simulink model "model_cnn"  (R2020a)
settings: Solver=VariableStepAuto  StartTime=0.0  StopTime=1e6/fs  RelTol=1e-3
PreLoadFcn:
  | setup_imports;
  | %dense2_numerictype = fixdt(1,18,10);
  | %conv1_numerictype = fixdt(1,18,21);
InitFcn:
  | % Intermediate signal dimensions
  | input_dim = [1, 2, 128];
  | layer1_dim = hInterConvLayerDims([1,3,1,64],input_dim,1); % dims : [C,H,W]
  | layer2_dim = hInterConvLayerDims([2,3,64,16],layer1_dim,1);% dims : [C,H,W]
  | layer3_dim = [1,128];
  | 
  | % Conv Layer 1 dimensions
  | conv1_dims = struct(...
  |     'input_dim',    input_dim,...       input_dim = C,H,W
  |     'filter_dim',   [1, 3, 1, 64],...  filter_dim = K,J,C,N
  |     'stride',       1,...
  |     'row_output',   3,...
  |     'output_dim',   layer1_dim);
  | 
  | % Conv Layer 2 dimensions
  | conv2_dims = struct(...
  |     'input_dim',    layer1_dim,...      input = C,H.W
  |     'filter_dim',   [2, 3, 64, 16],...  filter_dim = K,J,C,N
  |     'stride',       1,...
  |     'row_output',   2*3*64,...
  |     'output_dim',   layer2_dim);
  | 
  | % Dense Layer 1 dimensions
  | dense1_dims = struct(...
  |     'input_dim',    layer2_dim,...      input = C,H,W
  |     'weight_dim',   [1984, 128],...     weight_dim = H,W
  |     'output_dim',   layer3_dim);
  | 
  | % Load saved weights and input
  | setup_imports;
  | 
  | fs = 128e6;
  | fs_axi = 100e6;
  | R = 32;
values from neighbouring files (symbols this model uses):
  datatypeInput = X_test.numerictype    [setup_imports.m]
  gemm_wconv1 = fi(hInterleaveFilters(Wconv1),1,16)    [setup_imports.m]
  gemm_wconv2 = fi(hInterleaveFilters(Wconv2),1,16)    [setup_imports.m]
  wdense1 = fi(Wdense1,1,16)    [setup_imports.m]
  wdense2 = fi(Wdense2,1,16)    [setup_imports.m]
undefined symbols (not defined in the file or in its folder): ltehdlRAMinitPO2
libraries: hdlsllib x1022, dspsigops x3, dspsrcs4 x2
(part 1 of 23)
settings Model: SimulationMode=accelerator  Creator=andy  LastModifiedBy=andy
settings OptimizationCC: BlockReduction=off  ConditionallyExecuteInputs=off  DefaultParameterBehavior=Inlined
settings DebuggingCC: AlgebraicLoopMsg=error  ParameterOverflowMsg=none
settings HardwareCC: ProdBitPerPointer=32  ProdBitPerSizeT=32  ProdBitPerPtrDiffT=32  ProdLargestAtomicFloat=None  ProdIntDivRoundTo=Undefined  ProdEndianess=Unspecified  ProdWordSize=32  ProdHWDeviceType=ASIC/FPGA->ASIC/FPGA  TargetBitPerLong=64  TargetBitPerPointer=64  TargetBitPerSizeT=64  TargetBitPerPtrDiffT=64  TargetLongLongMode=on  TargetIntDivRoundTo=Zero  TargetEndianess=LittleEndian  TargetWordSize=64  TargetHWDeviceType=Custom Processor->MATLAB Host Computer  ProdEqTarget=off

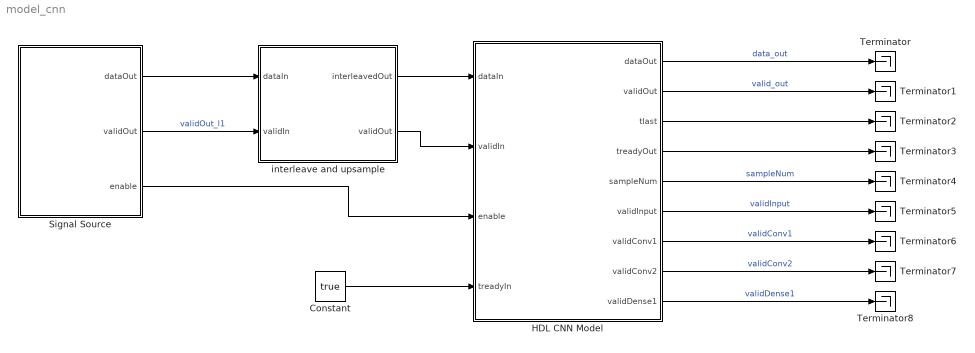
== system model_cnn ==
  Constant : Constant  Value=true  SampleTime=-1
  HDL CNN Model : Subsystem  TreatAsAtomicUnit=on
  Signal Source : Subsystem
  Terminator{,1..8} (9 alike) : Terminator
  interleave and upsample : Subsystem  TreatAsAtomicUnit=on
  wires:
  HDL CNN Model/1(dataOut) -> Terminator/1  "data_out"
  HDL CNN Model/2(validOut) -> Terminator1/1  "valid_out"
  HDL CNN Model/3(tlast) -> Terminator2/1
  Signal Source/3(enable) -> HDL CNN Model/3(enable)
  HDL CNN Model/4(treadyOut) -> Terminator3/1
  Constant/1 -> HDL CNN Model/4(treadyIn)
  HDL CNN Model/5(sampleNum) -> Terminator4/1  "sampleNum"
  HDL CNN Model/6(validInput) -> Terminator5/1  "validInput"
  HDL CNN Model/7(validConv1) -> Terminator6/1  "validConv1"
  HDL CNN Model/8(validConv2) -> Terminator7/1  "validConv2"
  HDL CNN Model/9(validDense1) -> Terminator8/1  "validDense1"
  interleave and upsample/1(interleavedOut) -> HDL CNN Model/1(dataIn)
  interleave and upsample/2(validOut) -> HDL CNN Model/2(validIn)
  Signal Source/1(dataOut) -> interleave and upsample/1(dataIn)
  Signal Source/2(validOut) -> interleave and upsample/2(validIn)  "validOut_l1"

== system model_cnn/HDL CNN Model ==
  note: Samples are being received:
      | Channel first, then Row, then Column
  dataIn : Inport
  validIn : Inport  Port=2
  enable : Inport  Port=3
  treadyIn : Inport  Port=4
  Collect Input into Bursts : Subsystem
  Constant : Constant  Value=7  OutDataTypeStr=fixdt(0,3)  SampleTime=-1
  Conv Layer 1 : Subsystem
  Conv Layer 2 : Subsystem
  Data Type Conversion1 : DataTypeConversion  OutDataTypeStr=single
  Delay{,1..11} (12 alike) : Delay  DelayLength=1
  Dense Layer 1 : Subsystem
  Dense Layer 2 : Subsystem
  Equal : RelationalOperator  Operator===  OutDataTypeStr=boolean  RndMeth=Simplest
  Float Typecast : FloatTypecast
  HDL Counter : hdlsllib/Sources/HDL Counter  CountType=Free running  CountInit=0  CountStep=1  CountMax=25  CountFromType=Initial value  CountFrom=0  CountResetPort=off  CountLoadPort=off  CountEnbPort=on  CountDirPort=off  CountDataType=Unsigned  CountWordLen=3  CountFracLen=0  CountSampTime=1
  Switch : Subsystem
  Terminator : Terminator
  always_ready : Constant  OutDataTypeStr=boolean  SampleTime=-1
  input switch : Subsystem
  dataOut : Outport
  validOut : Outport  Port=2
  tlast : Outport  Port=3
  treadyOut : Outport  Port=4
  sampleNum : Outport  Port=5
  validInput : Outport  Port=6
  validConv1 : Outport  Port=7
  validConv2 : Outport  Port=8
  validDense1 : Outport  Port=9
  wires:
  enable/1 -> Delay5/1
  validIn/1 -> validInput/1, Delay4/1
  Collect Input into Bursts/2(validOut) -> Conv Layer 1/2(validIn)  "validIn"
  Conv Layer 1/1(dataOut) -> Conv Layer 2/1(vectorIn)
  Conv Layer 1/2(validOut) -> validConv1/1, Conv Layer 2/2(validIn)  "validOut_l1"
  Collect Input into Bursts/1(dataOut) -> Conv Layer 1/1(dataIn)  "dataIn"
  Delay2/1 -> Conv Layer 1/3(enable)
  Delay1/1 -> Conv Layer 2/3(ready_nx_layer)
  Delay/1 -> Conv Layer 1/4(ready_nx_layer)
  Conv Layer 2/3(ready_prev) -> Delay/1  "ready_prev_l2"
  Conv Layer 2/1(vectorOut) -> Dense Layer 1/1(vectorIn)
  Conv Layer 2/2(validOut) -> validConv2/1, Dense Layer 1/2(validIn)  "validOut_l2"
  Dense Layer 1/3(ready_prev) -> Delay1/1
  Dense Layer 1/1(dataOut) -> Dense Layer 2/1(dataIn)
  Dense Layer 1/2(validOut) -> validDense1/1, Dense Layer 2/2(validIn)  "validOut_l3"
  Dense Layer 2/1(dataOut) -> Data Type Conversion1/1
  Dense Layer 2/2(validOut) -> Switch/1(validOut_l4)  "validOut_l4"
  dataIn/1 -> Delay3/1
  HDL Counter/1 -> Delay10/1, Equal/1  "count"
  Constant/1 -> Equal/2
  Equal/1 -> Delay8/1  "tlast"
  Data Type Conversion1/1 -> Float Typecast/1
  Float Typecast/1 -> Delay6/1
  Delay6/1 -> dataOut/1
  Delay7/1 -> validOut/1
  Delay8/1 -> tlast/1
  Delay4/1 -> input switch/1(validIn)
  Delay3/1 -> Collect Input into Bursts/1(dataIn)
  input switch/1(Out1) -> Collect Input into Bursts/2(validIn)
  Delay5/1 -> Delay2/1, Switch/2(ready), input switch/2(enable)
  Switch/1(Out1) -> HDL Counter/1, Delay7/1
  treadyIn/1 -> Delay9/1
  always_ready/1 -> Delay11/1
  Delay9/1 -> Terminator/1
  Delay11/1 -> treadyOut/1
  Delay10/1 -> sampleNum/1

== system model_cnn/Signal Source ==
  Bit Concat : hdlsllib/Logic and Bit Operations/Bit Concat  numInputs=2
  Complex to Real-Imag : ComplexToRealImag
  Constant1 : Constant  Value=true  SampleTime=R/fs
  Data Type Conversion1 : DataTypeConversion  OutDataTypeStr=boolean
  Repeat : dspsigops/Repeat  N=R  InputProcessing=Columns as channels (frame based)  RateOptions=Allow multirate processing  ic=0  mode=Unused parameter value
  Signal From Workspace : dspsrcs4/Signal From Workspace  X=dataIna  Ts=R/fs  nsamps=1  OutputAfterFinalValue=Setting to zero  ignoreOrWarnInputAndFrameLengths=off  OutputFrames=off
  Upsample1 : dspsigops/Upsample  N=R  phase=0  RateOptions=Allow multirate processing  ic=0  mode=Unused parameter value
  Upsample2 : dspsigops/Upsample  N=R  phase=0  RateOptions=Allow multirate processing  ic=0  mode=Unused parameter value
  valid samples : dspsrcs4/Signal From Workspace  X=valid  Ts=R/fs  nsamps=1  OutputAfterFinalValue=Setting to zero  ignoreOrWarnInputAndFrameLengths=off  OutputFrames=off
  dataOut : Outport
  validOut : Outport  Port=2
  enable : Outport  Port=3
  wires:
  Data Type Conversion1/1 -> Repeat/1  "ready"
  Constant1/1 -> Data Type Conversion1/1
  valid samples/1 -> Upsample2/1  "valid_in"
  Upsample1/1 -> dataOut/1
  Upsample2/1 -> validOut/1
  Repeat/1 -> enable/1
  Signal From Workspace/1 -> Complex to Real-Imag/1
  Complex to Real-Imag/2 -> Bit Concat/1
  Complex to Real-Imag/1 -> Bit Concat/2
  Bit Concat/1 -> Upsample1/1

== system model_cnn/interleave and upsample ==
  dataIn : Inport
  validIn : Inport  Port=2
  Bit Slice Imag : hdlsllib/Logic and Bit Operations/Bit Slice  lidx=31  ridx=16
      settings: SourceProductBaseCode=SL
  Bit Slice Real : hdlsllib/Logic and Bit Operations/Bit Slice  lidx=15  ridx=0
      settings: SourceProductBaseCode=SL
  Data Type Conversion2 : DataTypeConversion  OutDataTypeStr=fixdt(1,16,14)  ConvertRealWorld=Stored Integer (SI)
  Data Type Conversion3 : DataTypeConversion  OutDataTypeStr=fixdt(1,16,14)  ConvertRealWorld=Stored Integer (SI)
  Delay{1..5} (5 alike) : Delay  DelayLength=1
  Interleave IQ : Subsystem
  interleavedOut : Outport
  validOut : Outport  Port=2
  wires:
  Interleave IQ/1(interleavedOut) -> Delay4/1
  Bit Slice Imag/1 -> Data Type Conversion3/1
  Bit Slice Real/1 -> Data Type Conversion2/1
  dataIn/1 -> Bit Slice Imag/1, Bit Slice Real/1
  Data Type Conversion2/1 -> Delay3/1
  Data Type Conversion3/1 -> Delay1/1
  Interleave IQ/2(validOut) -> Delay5/1  "validIn"
  validIn/1 -> Delay2/1
  Delay3/1 -> Interleave IQ/1(Real)
  Delay1/1 -> Interleave IQ/2(Imag)
  Delay2/1 -> Interleave IQ/3(validIn)
  Delay4/1 -> interleavedOut/1
  Delay5/1 -> validOut/1

== system model_cnn/HDL CNN Model/Collect Input into Bursts ==
  dataIn : Inport
  validIn : Inport  Port=2
  Delay : Delay  DelayLength=1
  Delay1 : Delay  DelayLength=1
  NOT : Logic  Operator=NOT  IconShape=distinctive  AllPortsSameDT=off  OutDataTypeStr=boolean
  Ping Pong Buffer 0 : hdlsllib/HDL RAMs/Single Port RAM System  RAMType=Single port  WriteOutputValue=New data  RAMInitialValue=fi(zeros(1,512),datatypeInput)  SimulateUsing=Code generation
      settings: SourceProductBaseCode=SL
  Ping Pong Buffer 1 : hdlsllib/HDL RAMs/Single Port RAM System  RAMType=Single port  WriteOutputValue=New data  RAMInitialValue=fi(zeros(1,512),datatypeInput)  SimulateUsing=Code generation
      settings: SourceProductBaseCode=SL
  Ping Pong Buffer Controller : MATLAB Function  TreatAsAtomicUnit=on
  Switch : Switch  Criteria=u2 ~= 0
  dataOut : Outport
  validOut : Outport  Port=2
  wires:
  validIn/1 -> Ping Pong Buffer Controller/1(validIn)  "validIn"
  dataIn/1 -> Ping Pong Buffer 0/1, Ping Pong Buffer 1/1  "dataIn"
  Ping Pong Buffer 0/1 -> Switch/1  "pp0_out"
  Ping Pong Buffer 1/1 -> Switch/3  "pp1_out"
  Ping Pong Buffer Controller/3(bufferSelect) -> Delay/1  "bufferSelect"
  Delay/1 -> NOT/1
  Ping Pong Buffer Controller/6(validOut) -> Delay1/1  "validOut"
  Delay1/1 -> validOut/1
  Switch/1 -> dataOut/1  "dataOut"
  Ping Pong Buffer Controller/1(wr_en0) -> Ping Pong Buffer 0/3  "wr_en0"
  Ping Pong Buffer Controller/4(ram0_addr) -> Ping Pong Buffer 0/2  "ram0_addr"
  Ping Pong Buffer Controller/5(ram1_addr) -> Ping Pong Buffer 1/2  "ram1_addr"
  Ping Pong Buffer Controller/2(wr_en1) -> Ping Pong Buffer 1/3  "wr_en1"
  NOT/1 -> Switch/2  "bufferSelect"

== system model_cnn/HDL CNN Model/Conv Layer 1 ==
  dataIn : Inport
  validIn : Inport  Port=2
  enable : Inport  Port=3
  ready_nx_layer : Inport  Port=4
  Buffer and Sliding Window State Machine : MATLAB Function  TreatAsAtomicUnit=on
  Layer 1 Mat-Vec Multiplier : Subsystem
  Pipeline Delay{,1..6,9..10} (9 alike) : Delay  DelayLength=1
  RAM delay match : Delay  DelayLength=1
  ReLU : MATLAB Function  TreatAsAtomicUnit=on
  Simple Dual Port RAM System : hdlsllib/HDL RAMs/Simple Dual Port RAM System  RAMType=Simple dual port  WriteOutputValue=New data  RAMInitialValue=0  SimulateUsing=Code generation
      settings: SourceProductBaseCode=SL
  dataOut : Outport
  validOut : Outport  Port=2
  wires:
  Pipeline Delay10/1 -> Pipeline Delay5/1  "validIn"
  Pipeline Delay/1 -> Simple Dual Port RAM System/1  "dataIn"
  Buffer and Sliding Window State Machine/2(wr_en) -> Simple Dual Port RAM System/3  "wr_en"
  Buffer and Sliding Window State Machine/4(validOut) -> RAM delay match/1  "validOut"
  dataIn/1 -> Pipeline Delay/1
  Pipeline Delay4/1 -> Layer 1 Mat-Vec Multiplier/2(valid)  "gemm_sampleInValid"
  Simple Dual Port RAM System/1 -> Pipeline Delay3/1  "gemm_l1_out"
  validIn/1 -> Pipeline Delay1/1
  enable/1 -> Pipeline Delay2/1
  Pipeline Delay3/1 -> Layer 1 Mat-Vec Multiplier/1(dataIn)  "gemm_sampleIn"
  RAM delay match/1 -> Pipeline Delay4/1  "gemm_l1_valid"
  Pipeline Delay2/1 -> Buffer and Sliding Window State Machine/2(enable)
  ReLU/1(out) -> Pipeline Delay6/1  "act1_out"
  Buffer and Sliding Window State Machine/3(rd_addr) -> Simple Dual Port RAM System/4  "rd_addr"
  Layer 1 Mat-Vec Multiplier/2(validOut) -> Pipeline Delay10/1  "validOut_l1"
  Layer 1 Mat-Vec Multiplier/1(dataOut) -> Pipeline Delay9/1  "serialOut"
  Pipeline Delay1/1 -> Buffer and Sliding Window State Machine/1(validIn)  "validIn"
  Buffer and Sliding Window State Machine/1(wr_addr) -> Simple Dual Port RAM System/2  "wr_addr"
  ready_nx_layer/1 -> Buffer and Sliding Window State Machine/3(ready_nx_layer)
  Pipeline Delay5/1 -> validOut/1  "validIn"
  Pipeline Delay6/1 -> dataOut/1  "din"
  Pipeline Delay9/1 -> ReLU/1(in)  "din"

== system model_cnn/HDL CNN Model/Conv Layer 2 ==
  vectorIn : Inport
  validIn : Inport  Port=2
  ready_nx_layer : Inport  Port=3
  BRAM Storage Layer 2 : Subsystem
  Buffer and Sliding Window State Machine : MATLAB Function  TreatAsAtomicUnit=on
  Filter Matrix Multiplier1 : Subsystem
  Pipeline Delay{5..6,9..12} (6 alike) : Delay  DelayLength=1
  ReLU : MATLAB Function  TreatAsAtomicUnit=on
  Vector Slice Selection : Subsystem
  vectorOut : Outport
  validOut : Outport  Port=2
  ready_prev : Outport  Port=3
  wires:
  Buffer and Sliding Window State Machine/4(rd_row_idx) -> BRAM Storage Layer 2/5(rd_row_idx)
  Buffer and Sliding Window State Machine/2(wr_en) -> BRAM Storage Layer 2/3(wr_en)
  BRAM Storage Layer 2/2(validOut) -> Vector Slice Selection/2(validIn)  "gemm2_valid"
  Buffer and Sliding Window State Machine/1(wr_addr) -> BRAM Storage Layer 2/2(wr_addr)
  Buffer and Sliding Window State Machine/6(ready_prev) -> ready_prev/1  "ready_prev_l2"
  Filter Matrix Multiplier1/2(validOut) -> Pipeline Delay10/1
  Filter Matrix Multiplier1/1(vectorOut) -> Pipeline Delay9/1
  Pipeline Delay12/1 -> Filter Matrix Multiplier1/2(validIn)
  validIn/1 -> Buffer and Sliding Window State Machine/1(validIn)
  Pipeline Delay11/1 -> Filter Matrix Multiplier1/1(samplesIn)
  vectorIn/1 -> BRAM Storage Layer 2/1(vectorIn)
  BRAM Storage Layer 2/1(vectorOut) -> Vector Slice Selection/1(frameIn)  "gemm2_samples"
  Buffer and Sliding Window State Machine/3(rd_addr) -> BRAM Storage Layer 2/4(rd_addr)
  Buffer and Sliding Window State Machine/5(validOut) -> BRAM Storage Layer 2/6(validIn)
  Pipeline Delay9/1 -> ReLU/1(in)  "din"
  Pipeline Delay10/1 -> Pipeline Delay5/1  "validIn"
  ReLU/1(out) -> Pipeline Delay6/1
  Pipeline Delay5/1 -> validOut/1
  Pipeline Delay6/1 -> vectorOut/1
  ready_nx_layer/1 -> Buffer and Sliding Window State Machine/2(ready_nx_layer)
  Vector Slice Selection/1(frameOut) -> Pipeline Delay11/1
  Vector Slice Selection/2(validOut) -> Pipeline Delay12/1

== system model_cnn/HDL CNN Model/Dense Layer 1 ==
  vectorIn : Inport
  validIn : Inport  Port=2
  BRAM Storage Layer 2 : Subsystem
  Dense Layer 1 : Subsystem
  Output Buffer1 : MATLAB Function  TreatAsAtomicUnit=on
  Pipeline Delay{1..2,5..6} (4 alike) : Delay  DelayLength=1
  ReLU 3 : MATLAB Function  TreatAsAtomicUnit=on
  Sample Storage Buffer1 : MATLAB Function  TreatAsAtomicUnit=on
  Terminator : Terminator
  dataOut : Outport
  validOut : Outport  Port=2
  ready_prev : Outport  Port=3
  wires:
  Dense Layer 1/2(validOut) -> Output Buffer1/2(validIn)  "validOut_l3"
  Pipeline Delay1/1 -> Dense Layer 1/1(dataIn)  "bias2_out_samples"
  Output Buffer1/3(done) -> Terminator/1  "done"
  validIn/1 -> Sample Storage Buffer1/1(validIn)
  BRAM Storage Layer 2/1(sampleOut) -> Pipeline Delay1/1  "out2_samples"
  Sample Storage Buffer1/5(validOut) -> BRAM Storage Layer 2/6(validIn)
  Sample Storage Buffer1/2(wr_en) -> BRAM Storage Layer 2/3(wr_en)
  vectorIn/1 -> BRAM Storage Layer 2/1(vectorIn)
  Sample Storage Buffer1/6(ready_prev) -> ready_prev/1
  Pipeline Delay6/1 -> validOut/1  "bias3_out_valid"
  Pipeline Delay2/1 -> Dense Layer 1/2(valid)  "bias2_out_valid"
  Sample Storage Buffer1/4(rd_row_idx) -> BRAM Storage Layer 2/5(rd_row_idx)  "rd_row_idx"
  Sample Storage Buffer1/1(wr_addr) -> BRAM Storage Layer 2/2(wr_addr)
  Pipeline Delay5/1 -> ReLU 3/1(in)  "bias3_out_samples"
  BRAM Storage Layer 2/2(validOut) -> Pipeline Delay2/1  "out2_valid"
  Output Buffer1/2(validOut) -> Pipeline Delay6/1  "samplesValid"
  Sample Storage Buffer1/3(rd_addr) -> BRAM Storage Layer 2/4(rd_addr)  "rd_addr"
  Dense Layer 1/1(dataOut) -> Output Buffer1/1(vectorIn)  "samplesOut"
  Output Buffer1/1(samplesOut) -> Pipeline Delay5/1  "samplesOut"
  ReLU 3/1(out) -> dataOut/1  "din"

== system model_cnn/HDL CNN Model/Dense Layer 2 ==
  dataIn : Inport
  validIn : Inport  Port=2
  Dense Layer 2 : Subsystem
  Output Buffer3 : MATLAB Function  TreatAsAtomicUnit=on
  Pipeline Delay{7..8,13..14} (4 alike) : Delay  DelayLength=1
  Terminator1 : Terminator
  dataOut : Outport
  validOut : Outport  Port=2
  wires:
  Pipeline Delay7/1 -> Pipeline Delay13/1  "bias4_out_samples"
  dataIn/1 -> Dense Layer 2/1(dataIn)
  validIn/1 -> Dense Layer 2/2(validIn)
  Output Buffer3/3(done) -> Terminator1/1  "done"
  Output Buffer3/1(samplesOut) -> Pipeline Delay7/1  "samplesOut"
  Pipeline Delay14/1 -> validOut/1
  Pipeline Delay13/1 -> dataOut/1
  Dense Layer 2/2(validOut) -> Output Buffer3/2(validIn)  "validOut_l4"
  Output Buffer3/2(validOut) -> Pipeline Delay8/1  "samplesValid"
  Dense Layer 2/1(dataOut) -> Output Buffer3/1(vectorIn)  "samplesOut"
  Pipeline Delay8/1 -> Pipeline Delay14/1  "bias4_out_valid"

== system model_cnn/HDL CNN Model/Switch ==
  validOut_l4 : Inport
  ready : Inport  Port=2
  Constant : Constant  Value=false  SampleTime=-1
  Switch : Switch  Criteria=u2 > Threshold  Threshold=0.5
  Out1 : Outport
  wires:
  validOut_l4/1 -> Switch/1
  ready/1 -> Switch/2
  Constant/1 -> Switch/3
  Switch/1 -> Out1/1

== system model_cnn/HDL CNN Model/input switch ==
  validIn : Inport
  enable : Inport  Port=2
  Constant : Constant  Value=false  SampleTime=-1
  Switch : Switch  Criteria=u2 > Threshold  Threshold=0.5
  Out1 : Outport
  wires:
  validIn/1 -> Switch/1
  enable/1 -> Switch/2
  Constant/1 -> Switch/3
  Switch/1 -> Out1/1

== system model_cnn/interleave and upsample/Interleave IQ ==
  Real : Inport
  Imag : Inport  Port=2
  validIn : Inport  Port=3
  Add : Sum
  Delay : Delay  DelayLength=1
  Delay1 : Delay  DelayLength=1
  OR : Logic  Operator=OR  IconShape=distinctive  AllPortsSameDT=off  OutDataTypeStr=boolean
  interleavedOut : Outport
  validOut : Outport  Port=2
  wires:
  Imag/1 -> Delay/1
  Delay/1 -> Add/2
  Add/1 -> interleavedOut/1
  Real/1 -> Add/1
  validIn/1 -> Delay1/1, OR/1
  Delay1/1 -> OR/2
  OR/1 -> validOut/1

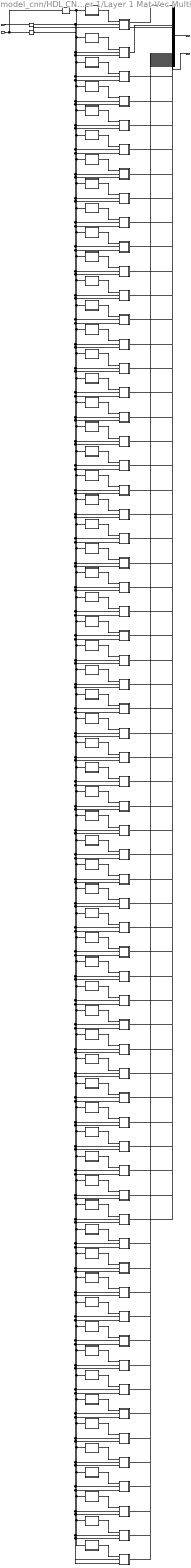
== system model_cnn/HDL CNN Model/Conv Layer 1/Layer 1 Mat-Vec Multiplier ==
  dataIn : Inport
  valid : Inport  Port=2
  Delay : Delay  DelayLength=1
  Delay1 : Delay  DelayLength=1
  HDL Counter : hdlsllib/Sources/HDL Counter  CountType=Count limited  CountInit=0  CountStep=1  CountMax=3-1  CountFromType=Initial value  CountFrom=0  CountResetPort=off  CountLoadPort=off  CountEnbPort=on  CountDirPort=off  CountDataType=Unsigned  CountWordLen=ceil(log2(3))  CountFracLen=0  CountSampTime=1
  Vector Concatenate : Concatenate  NumInputs=64
  Weight Storage 0 : Subsystem  mask{dim=1}
      mask prompts: dim "Filter Selection"
  Weight Storage1 : Subsystem  mask{dim=2}
      mask prompts: dim "Filter Selection"
  Weight Storage10 : Subsystem  mask{dim=11}
      mask prompts: dim "Filter Selection"
  Weight Storage11 : Subsystem  mask{dim=12}
      mask prompts: dim "Filter Selection"
  Weight Storage12 : Subsystem  mask{dim=13}
      mask prompts: dim "Filter Selection"
  Weight Storage13 : Subsystem  mask{dim=14}
      mask prompts: dim "Filter Selection"
  Weight Storage14 : Subsystem  mask{dim=15}
      mask prompts: dim "Filter Selection"
  Weight Storage15 : Subsystem  mask{dim=16}
      mask prompts: dim "Filter Selection"
  Weight Storage16 : Subsystem  mask{dim=17}
      mask prompts: dim "Filter Selection"
  Weight Storage17 : Subsystem  mask{dim=18}
      mask prompts: dim "Filter Selection"
  Weight Storage18 : Subsystem  mask{dim=19}
      mask prompts: dim "Filter Selection"
  Weight Storage19 : Subsystem  mask{dim=20}
      mask prompts: dim "Filter Selection"
  Weight Storage2 : Subsystem  mask{dim=3}
      mask prompts: dim "Filter Selection"
  Weight Storage20 : Subsystem  mask{dim=21}
      mask prompts: dim "Filter Selection"
  Weight Storage21 : Subsystem  mask{dim=22}
      mask prompts: dim "Filter Selection"
  Weight Storage22 : Subsystem  mask{dim=23}
      mask prompts: dim "Filter Selection"
  Weight Storage23 : Subsystem  mask{dim=24}
      mask prompts: dim "Filter Selection"
  Weight Storage24 : Subsystem  mask{dim=25}
      mask prompts: dim "Filter Selection"
  Weight Storage25 : Subsystem  mask{dim=26}
      mask prompts: dim "Filter Selection"
  Weight Storage26 : Subsystem  mask{dim=27}
      mask prompts: dim "Filter Selection"
  Weight Storage27 : Subsystem  mask{dim=28}
      mask prompts: dim "Filter Selection"
  Weight Storage28 : Subsystem  mask{dim=29}
      mask prompts: dim "Filter Selection"
  Weight Storage29 : Subsystem  mask{dim=30}
      mask prompts: dim "Filter Selection"
  Weight Storage3 : Subsystem  mask{dim=4}
      mask prompts: dim "Filter Selection"
  Weight Storage30 : Subsystem  mask{dim=31}
      mask prompts: dim "Filter Selection"
  Weight Storage31 : Subsystem  mask{dim=32}
      mask prompts: dim "Filter Selection"
  Weight Storage32 : Subsystem  mask{dim=33}
      mask prompts: dim "Filter Selection"
  Weight Storage33 : Subsystem  mask{dim=34}
      mask prompts: dim "Filter Selection"
  Weight Storage34 : Subsystem  mask{dim=35}
      mask prompts: dim "Filter Selection"
  Weight Storage35 : Subsystem  mask{dim=36}
      mask prompts: dim "Filter Selection"
  Weight Storage36 : Subsystem  mask{dim=37}
      mask prompts: dim "Filter Selection"
  Weight Storage37 : Subsystem  mask{dim=38}
      mask prompts: dim "Filter Selection"
  Weight Storage38 : Subsystem  mask{dim=39}
      mask prompts: dim "Filter Selection"
  Weight Storage39 : Subsystem  mask{dim=40}
      mask prompts: dim "Filter Selection"
  Weight Storage4 : Subsystem  mask{dim=5}
      mask prompts: dim "Filter Selection"
  Weight Storage40 : Subsystem  mask{dim=41}
      mask prompts: dim "Filter Selection"
  Weight Storage41 : Subsystem  mask{dim=42}
      mask prompts: dim "Filter Selection"
  Weight Storage42 : Subsystem  mask{dim=43}
      mask prompts: dim "Filter Selection"
  Weight Storage43 : Subsystem  mask{dim=44}
      mask prompts: dim "Filter Selection"
  Weight Storage44 : Subsystem  mask{dim=45}
      mask prompts: dim "Filter Selection"
  Weight Storage45 : Subsystem  mask{dim=46}
      mask prompts: dim "Filter Selection"
  Weight Storage46 : Subsystem  mask{dim=47}
      mask prompts: dim "Filter Selection"
  Weight Storage47 : Subsystem  mask{dim=48}
      mask prompts: dim "Filter Selection"
  Weight Storage48 : Subsystem  mask{dim=49}
      mask prompts: dim "Filter Selection"
  Weight Storage49 : Subsystem  mask{dim=50}
      mask prompts: dim "Filter Selection"
  Weight Storage5 : Subsystem  mask{dim=6}
      mask prompts: dim "Filter Selection"
  Weight Storage50 : Subsystem  mask{dim=51}
      mask prompts: dim "Filter Selection"
  Weight Storage51 : Subsystem  mask{dim=52}
      mask prompts: dim "Filter Selection"
  Weight Storage52 : Subsystem  mask{dim=53}
      mask prompts: dim "Filter Selection"
  Weight Storage53 : Subsystem  mask{dim=54}
      mask prompts: dim "Filter Selection"
  Weight Storage54 : Subsystem  mask{dim=55}
      mask prompts: dim "Filter Selection"
  Weight Storage55 : Subsystem  mask{dim=56}
      mask prompts: dim "Filter Selection"
  Weight Storage56 : Subsystem  mask{dim=57}
      mask prompts: dim "Filter Selection"
  Weight Storage57 : Subsystem  mask{dim=58}
      mask prompts: dim "Filter Selection"
  Weight Storage58 : Subsystem  mask{dim=59}
      mask prompts: dim "Filter Selection"
  Weight Storage59 : Subsystem  mask{dim=60}
      mask prompts: dim "Filter Selection"
  Weight Storage6 : Subsystem  mask{dim=7}
      mask prompts: dim "Filter Selection"
  Weight Storage60 : Subsystem  mask{dim=61}
      mask prompts: dim "Filter Selection"
  Weight Storage61 : Subsystem  mask{dim=62}
      mask prompts: dim "Filter Selection"
  Weight Storage62 : Subsystem  mask{dim=63}
      mask prompts: dim "Filter Selection"
  Weight Storage63 : Subsystem  mask{dim=64}
      mask prompts: dim "Filter Selection"
  Weight Storage7 : Subsystem  mask{dim=8}
      mask prompts: dim "Filter Selection"
  Weight Storage8 : Subsystem  mask{dim=9}
      mask prompts: dim "Filter Selection"
  Weight Storage9 : Subsystem  mask{dim=10}
      mask prompts: dim "Filter Selection"
  adder 0 : Subsystem
  adder1 : Subsystem
  adder10 : Subsystem
  adder11 : Subsystem
  adder12 : Subsystem
  adder13 : Subsystem
  adder14 : Subsystem
  adder15 : Subsystem
  adder16 : Subsystem
  adder17 : Subsystem
  adder18 : Subsystem
  adder19 : Subsystem
  adder2 : Subsystem
  adder20 : Subsystem
  adder21 : Subsystem
  adder22 : Subsystem
  adder23 : Subsystem
  adder24 : Subsystem
  adder25 : Subsystem
  adder26 : Subsystem
  adder27 : Subsystem
  adder28 : Subsystem
  adder29 : Subsystem
  adder3 : Subsystem
  adder30 : Subsystem
  adder31 : Subsystem
  adder32 : Subsystem
  adder33 : Subsystem
  adder34 : Subsystem
  adder35 : Subsystem
  adder36 : Subsystem
  adder37 : Subsystem
  adder38 : Subsystem
  adder39 : Subsystem
  adder4 : Subsystem
  adder40 : Subsystem
  adder41 : Subsystem
  adder42 : Subsystem
  adder43 : Subsystem
  adder44 : Subsystem
  adder45 : Subsystem
  adder46 : Subsystem
  adder47 : Subsystem
  adder48 : Subsystem
  adder49 : Subsystem
  adder5 : Subsystem
  adder50 : Subsystem
  adder51 : Subsystem
  adder52 : Subsystem
  adder53 : Subsystem
  adder54 : Subsystem
  adder55 : Subsystem
  adder56 : Subsystem
  adder57 : Subsystem
  adder58 : Subsystem
  adder59 : Subsystem
  adder6 : Subsystem
  adder60 : Subsystem
  adder61 : Subsystem
  adder62 : Subsystem
  adder63 : Subsystem
  adder7 : Subsystem
  adder8 : Subsystem
  adder9 : Subsystem
  dataOut : Outport
  validOut : Outport  Port=2
  wires:
  dataIn/1 -> Delay/1
  valid/1 -> Delay1/1, HDL Counter/1
  HDL Counter/1 -> Weight Storage62/1(count_Weights), Weight Storage63/1(count_Weights), Weight Storage61/1(count_Weights), Weight Storage60/1(count_Weights), Weight Storage59/1(count_Weights), Weight Storage58/1(count_Weights), Weight Storage57/1(count_Weights), Weight Storage56/1(count_Weights), Weight Storage55/1(count_Weights), Weight Storage54/1(count_Weights), Weight Storage53/1(count_Weights), Weight Storage52/1(count_Weights), Weight Storage51/1(count_Weights), Weight Storage50/1(count_Weights), Weight Storage49/1(count_Weights), Weight Storage48/1(count_Weights), Weight Storage47/1(count_Weights), Weight Storage46/1(count_Weights), Weight Storage45/1(count_Weights), Weight Storage44/1(count_Weights), Weight Storage43/1(count_Weights), Weight Storage42/1(count_Weights), Weight Storage41/1(count_Weights), Weight Storage40/1(count_Weights), Weight Storage39/1(count_Weights), Weight Storage38/1(count_Weights), Weight Storage37/1(count_Weights), Weight Storage36/1(count_Weights), Weight Storage35/1(count_Weights), Weight Storage34/1(count_Weights), Weight Storage33/1(count_Weights), Weight Storage32/1(count_Weights), Weight Storage31/1(count_Weights), Weight Storage30/1(count_Weights), Weight Storage29/1(count_Weights), Weight Storage28/1(count_Weights), Weight Storage27/1(count_Weights), Weight Storage26/1(count_Weights), Weight Storage25/1(count_Weights), Weight Storage24/1(count_Weights), Weight Storage23/1(count_Weights), Weight Storage22/1(count_Weights), Weight Storage21/1(count_Weights), Weight Storage20/1(count_Weights), Weight Storage19/1(count_Weights), Weight Storage18/1(count_Weights), Weight Storage17/1(count_Weights), Weight Storage16/1(count_Weights), Weight Storage15/1(count_Weights), Weight Storage14/1(count_Weights), Weight Storage13/1(count_Weights), Weight Storage12/1(count_Weights), Weight Storage11/1(count_Weights), Weight Storage10/1(count_Weights), Weight Storage9/1(count_Weights), Weight Storage8/1(count_Weights), Weight Storage7/1(count_Weights), Weight Storage6/1(count_Weights), Weight Storage5/1(count_Weights), Weight Storage4/1(count_Weights), Weight Storage3/1(count_Weights), Weight Storage2/1(count_Weights), Weight Storage1/1(count_Weights), Weight Storage 0/1(count_Weights)  "count_Weights"
  Weight Storage 0/1(Out1) -> adder 0/1(In1)
  Delay/1 -> adder62/2(In2), adder63/2(In2), adder61/2(In2), adder60/2(In2), adder59/2(In2), adder58/2(In2), adder57/2(In2), adder56/2(In2), adder55/2(In2), adder54/2(In2), adder53/2(In2), adder52/2(In2), adder51/2(In2), adder50/2(In2), adder49/2(In2), adder48/2(In2), adder47/2(In2), adder46/2(In2), adder45/2(In2), adder44/2(In2), adder43/2(In2), adder42/2(In2), adder41/2(In2), adder40/2(In2), adder39/2(In2), adder38/2(In2), adder37/2(In2), adder36/2(In2), adder35/2(In2), adder34/2(In2), adder33/2(In2), adder32/2(In2), adder31/2(In2), adder30/2(In2), adder29/2(In2), adder28/2(In2), adder27/2(In2), adder26/2(In2), adder25/2(In2), adder24/2(In2), adder23/2(In2), adder22/2(In2), adder21/2(In2), adder20/2(In2), adder19/2(In2), adder18/2(In2), adder17/2(In2), adder16/2(In2), adder15/2(In2), adder14/2(In2), adder13/2(In2), adder12/2(In2), adder11/2(In2), adder10/2(In2), adder9/2(In2), adder8/2(In2), adder7/2(In2), adder6/2(In2), adder5/2(In2), adder4/2(In2), adder3/2(In2), adder2/2(In2), adder1/2(In2), adder 0/2(In2)
  Delay1/1 -> adder62/3(In3), adder63/3(In3), adder61/3(In3), adder60/3(In3), adder59/3(In3), adder58/3(In3), adder57/3(In3), adder56/3(In3), adder55/3(In3), adder54/3(In3), adder53/3(In3), adder52/3(In3), adder51/3(In3), adder50/3(In3), adder49/3(In3), adder48/3(In3), adder47/3(In3), adder46/3(In3), adder45/3(In3), adder44/3(In3), adder43/3(In3), adder42/3(In3), adder41/3(In3), adder40/3(In3), adder39/3(In3), adder38/3(In3), adder37/3(In3), adder36/3(In3), adder35/3(In3), adder34/3(In3), adder33/3(In3), adder32/3(In3), adder31/3(In3), adder30/3(In3), adder29/3(In3), adder28/3(In3), adder27/3(In3), adder26/3(In3), adder25/3(In3), adder24/3(In3), adder23/3(In3), adder22/3(In3), adder21/3(In3), adder20/3(In3), adder19/3(In3), adder18/3(In3), adder17/3(In3), adder16/3(In3), adder15/3(In3), adder14/3(In3), adder13/3(In3), adder12/3(In3), adder11/3(In3), adder10/3(In3), adder9/3(In3), adder8/3(In3), adder7/3(In3), adder6/3(In3), adder5/3(In3), adder4/3(In3), adder3/3(In3), adder2/3(In3), adder1/3(In3), adder 0/3(In3)
  adder 0/1(dataOut) -> Vector Concatenate/1
  Vector Concatenate/1 -> dataOut/1
  adder 0/2(validOut) -> validOut/1
  Weight Storage1/1(Out1) -> adder1/1(In1)
  adder1/1(dataOut) -> Vector Concatenate/2
  Weight Storage2/1(Out1) -> adder2/1(In1)
  adder2/1(dataOut) -> Vector Concatenate/3
  Weight Storage3/1(Out1) -> adder3/1(In1)
  adder3/1(dataOut) -> Vector Concatenate/4
  Weight Storage4/1(Out1) -> adder4/1(In1)
  adder4/1(dataOut) -> Vector Concatenate/5
  Weight Storage5/1(Out1) -> adder5/1(In1)
  adder5/1(dataOut) -> Vector Concatenate/6
  Weight Storage6/1(Out1) -> adder6/1(In1)
  adder6/1(dataOut) -> Vector Concatenate/7
  Weight Storage7/1(Out1) -> adder7/1(In1)
  adder7/1(dataOut) -> Vector Concatenate/8
  Weight Storage8/1(Out1) -> adder8/1(In1)
  adder8/1(dataOut) -> Vector Concatenate/9
  Weight Storage9/1(Out1) -> adder9/1(In1)
  adder9/1(dataOut) -> Vector Concatenate/10
  Weight Storage10/1(Out1) -> adder10/1(In1)
  adder10/1(dataOut) -> Vector Concatenate/11
  Weight Storage11/1(Out1) -> adder11/1(In1)
  adder11/1(dataOut) -> Vector Concatenate/12
  Weight Storage12/1(Out1) -> adder12/1(In1)
  adder12/1(dataOut) -> Vector Concatenate/13
  Weight Storage13/1(Out1) -> adder13/1(In1)
  adder13/1(dataOut) -> Vector Concatenate/14
  Weight Storage14/1(Out1) -> adder14/1(In1)
  adder14/1(dataOut) -> Vector Concatenate/15
  Weight Storage15/1(Out1) -> adder15/1(In1)
  adder15/1(dataOut) -> Vector Concatenate/16
  Weight Storage16/1(Out1) -> adder16/1(In1)
  adder16/1(dataOut) -> Vector Concatenate/17
  Weight Storage17/1(Out1) -> adder17/1(In1)
  adder17/1(dataOut) -> Vector Concatenate/18
  Weight Storage18/1(Out1) -> adder18/1(In1)
  adder18/1(dataOut) -> Vector Concatenate/19
  Weight Storage19/1(Out1) -> adder19/1(In1)
  adder19/1(dataOut) -> Vector Concatenate/20
  Weight Storage20/1(Out1) -> adder20/1(In1)
  adder20/1(dataOut) -> Vector Concatenate/21
  Weight Storage21/1(Out1) -> adder21/1(In1)
  adder21/1(dataOut) -> Vector Concatenate/22
  Weight Storage22/1(Out1) -> adder22/1(In1)
  adder22/1(dataOut) -> Vector Concatenate/23
  Weight Storage23/1(Out1) -> adder23/1(In1)
  adder23/1(dataOut) -> Vector Concatenate/24
  Weight Storage24/1(Out1) -> adder24/1(In1)
  adder24/1(dataOut) -> Vector Concatenate/25
  Weight Storage25/1(Out1) -> adder25/1(In1)
  adder25/1(dataOut) -> Vector Concatenate/26
  Weight Storage26/1(Out1) -> adder26/1(In1)
  adder26/1(dataOut) -> Vector Concatenate/27
  Weight Storage27/1(Out1) -> adder27/1(In1)
  adder27/1(dataOut) -> Vector Concatenate/28
  Weight Storage28/1(Out1) -> adder28/1(In1)
  adder28/1(dataOut) -> Vector Concatenate/29
  Weight Storage29/1(Out1) -> adder29/1(In1)
  adder29/1(dataOut) -> Vector Concatenate/30
  Weight Storage30/1(Out1) -> adder30/1(In1)
  adder30/1(dataOut) -> Vector Concatenate/31
  Weight Storage31/1(Out1) -> adder31/1(In1)
  adder31/1(dataOut) -> Vector Concatenate/32
  Weight Storage32/1(Out1) -> adder32/1(In1)
  adder32/1(dataOut) -> Vector Concatenate/33
  Weight Storage33/1(Out1) -> adder33/1(In1)
  adder33/1(dataOut) -> Vector Concatenate/34
  Weight Storage34/1(Out1) -> adder34/1(In1)
  adder34/1(dataOut) -> Vector Concatenate/35
  Weight Storage35/1(Out1) -> adder35/1(In1)
  adder35/1(dataOut) -> Vector Concatenate/36
  Weight Storage36/1(Out1) -> adder36/1(In1)
  adder36/1(dataOut) -> Vector Concatenate/37
  Weight Storage37/1(Out1) -> adder37/1(In1)
  adder37/1(dataOut) -> Vector Concatenate/38
  Weight Storage38/1(Out1) -> adder38/1(In1)
  adder38/1(dataOut) -> Vector Concatenate/39
  Weight Storage39/1(Out1) -> adder39/1(In1)
  adder39/1(dataOut) -> Vector Concatenate/40
  Weight Storage40/1(Out1) -> adder40/1(In1)
  adder40/1(dataOut) -> Vector Concatenate/41
  Weight Storage41/1(Out1) -> adder41/1(In1)
  adder41/1(dataOut) -> Vector Concatenate/42
  Weight Storage42/1(Out1) -> adder42/1(In1)
  adder42/1(dataOut) -> Vector Concatenate/43
  Weight Storage43/1(Out1) -> adder43/1(In1)
  adder43/1(dataOut) -> Vector Concatenate/44
  Weight Storage44/1(Out1) -> adder44/1(In1)
  adder44/1(dataOut) -> Vector Concatenate/45
  Weight Storage45/1(Out1) -> adder45/1(In1)
  adder45/1(dataOut) -> Vector Concatenate/46
  Weight Storage46/1(Out1) -> adder46/1(In1)
  adder46/1(dataOut) -> Vector Concatenate/47
  Weight Storage47/1(Out1) -> adder47/1(In1)
  adder47/1(dataOut) -> Vector Concatenate/48
  Weight Storage48/1(Out1) -> adder48/1(In1)
  adder48/1(dataOut) -> Vector Concatenate/49
  Weight Storage49/1(Out1) -> adder49/1(In1)
  adder49/1(dataOut) -> Vector Concatenate/50
  Weight Storage50/1(Out1) -> adder50/1(In1)
  adder50/1(dataOut) -> Vector Concatenate/51
  Weight Storage51/1(Out1) -> adder51/1(In1)
  adder51/1(dataOut) -> Vector Concatenate/52
  Weight Storage52/1(Out1) -> adder52/1(In1)
  adder52/1(dataOut) -> Vector Concatenate/53
  Weight Storage53/1(Out1) -> adder53/1(In1)
  adder53/1(dataOut) -> Vector Concatenate/54
  Weight Storage54/1(Out1) -> adder54/1(In1)
  adder54/1(dataOut) -> Vector Concatenate/55
  Weight Storage55/1(Out1) -> adder55/1(In1)
  adder55/1(dataOut) -> Vector Concatenate/56
  Weight Storage56/1(Out1) -> adder56/1(In1)
  adder56/1(dataOut) -> Vector Concatenate/57
  Weight Storage57/1(Out1) -> adder57/1(In1)
  adder57/1(dataOut) -> Vector Concatenate/58
  Weight Storage58/1(Out1) -> adder58/1(In1)
  adder58/1(dataOut) -> Vector Concatenate/59
  Weight Storage59/1(Out1) -> adder59/1(In1)
  adder59/1(dataOut) -> Vector Concatenate/60
  Weight Storage60/1(Out1) -> adder60/1(In1)
  adder60/1(dataOut) -> Vector Concatenate/61
  Weight Storage61/1(Out1) -> adder61/1(In1)
  adder61/1(dataOut) -> Vector Concatenate/62
  Weight Storage62/1(Out1) -> adder62/1(In1)
  adder62/1(dataOut) -> Vector Concatenate/63
  Weight Storage63/1(Out1) -> adder63/1(In1)
  adder63/1(dataOut) -> Vector Concatenate/64

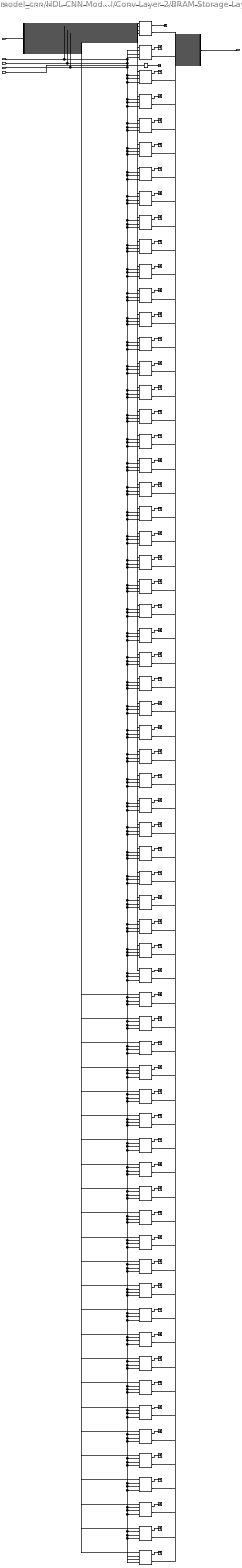
== system model_cnn/HDL CNN Model/Conv Layer 2/BRAM Storage Layer 2 ==
  vectorIn : Inport
  wr_addr : Inport  Port=2
  wr_en : Inport  Port=3
  rd_addr : Inport  Port=4
  rd_row_idx : Inport  Port=5
  validIn : Inport  Port=6
  Delay : Delay  DelayLength=1
  Delay1 : Delay  DelayLength=1
  Demux : Demux  Outputs=64
  RAM 0 : hdlsllib/HDL RAMs/Dual Port RAM System  RAMType=Dual port  WriteOutputValue=New data  RAMInitialValue=0  SimulateUsing=Code generation
      settings: SourceProductBaseCode=SL
  RAM{1..63} (63 alike) : hdlsllib/HDL RAMs/Dual Port RAM System  RAMType=Dual port  WriteOutputValue=New data  RAMInitialValue=0  SimulateUsing=Code generation
      settings: SourceProductBaseCode=SL
  Terminator : Terminator
  Terminator1 : Terminator
  Vector Concatenate : Concatenate  NumInputs=64
  term_{2..64} (63 alike) : Terminator
  vectorOut : Outport
  validOut : Outport  Port=2
  wires:
  vectorIn/1 -> Demux/1
  Demux/1 -> RAM 0/1
  Vector Concatenate/1 -> vectorOut/1
  wr_addr/1 -> RAM62/2, RAM63/2, RAM61/2, RAM60/2, RAM59/2, RAM58/2, RAM57/2, RAM56/2, RAM55/2, RAM54/2, RAM53/2, RAM52/2, RAM51/2, RAM50/2, RAM49/2, RAM48/2, RAM47/2, RAM46/2, RAM45/2, RAM44/2, RAM43/2, RAM42/2, RAM41/2, RAM40/2, RAM39/2, RAM38/2, RAM37/2, RAM36/2, RAM35/2, RAM34/2, RAM33/2, RAM32/2, RAM31/2, RAM30/2, RAM29/2, RAM28/2, RAM27/2, RAM26/2, RAM25/2, RAM24/2, RAM23/2, RAM22/2, RAM21/2, RAM20/2, RAM19/2, RAM18/2, RAM17/2, RAM16/2, RAM15/2, RAM14/2, RAM13/2, RAM12/2, RAM11/2, RAM10/2, RAM9/2, RAM8/2, RAM7/2, RAM6/2, RAM5/2, RAM4/2, RAM3/2, RAM2/2, RAM1/2, RAM 0/2
  RAM 0/1 -> Terminator/1
  RAM 0/2 -> Vector Concatenate/1
  validIn/1 -> Delay/1
  Delay/1 -> validOut/1
  wr_en/1 -> RAM62/3, RAM63/3, RAM61/3, RAM60/3, RAM59/3, RAM58/3, RAM57/3, RAM56/3, RAM55/3, RAM54/3, RAM53/3, RAM52/3, RAM51/3, RAM50/3, RAM49/3, RAM48/3, RAM47/3, RAM46/3, RAM45/3, RAM44/3, RAM43/3, RAM42/3, RAM41/3, RAM40/3, RAM39/3, RAM38/3, RAM37/3, RAM36/3, RAM35/3, RAM34/3, RAM33/3, RAM32/3, RAM31/3, RAM30/3, RAM29/3, RAM28/3, RAM27/3, RAM26/3, RAM25/3, RAM24/3, RAM23/3, RAM22/3, RAM21/3, RAM20/3, RAM19/3, RAM18/3, RAM17/3, RAM16/3, RAM15/3, RAM14/3, RAM13/3, RAM12/3, RAM11/3, RAM10/3, RAM9/3, RAM8/3, RAM7/3, RAM6/3, RAM5/3, RAM4/3, RAM3/3, RAM2/3, RAM1/3, RAM 0/3  "wr_en"
  rd_addr/1 -> RAM62/4, RAM63/4, RAM61/4, RAM60/4, RAM59/4, RAM58/4, RAM57/4, RAM56/4, RAM55/4, RAM54/4, RAM53/4, RAM52/4, RAM51/4, RAM50/4, RAM49/4, RAM48/4, RAM47/4, RAM46/4, RAM45/4, RAM44/4, RAM43/4, RAM42/4, RAM41/4, RAM40/4, RAM39/4, RAM38/4, RAM37/4, RAM36/4, RAM35/4, RAM34/4, RAM33/4, RAM32/4, RAM31/4, RAM30/4, RAM29/4, RAM28/4, RAM27/4, RAM26/4, RAM25/4, RAM24/4, RAM23/4, RAM22/4, RAM21/4, RAM20/4, RAM19/4, RAM18/4, RAM17/4, RAM16/4, RAM15/4, RAM14/4, RAM13/4, RAM12/4, RAM11/4, RAM10/4, RAM9/4, RAM8/4, RAM7/4, RAM6/4, RAM5/4, RAM4/4, RAM3/4, RAM2/4, RAM1/4, RAM 0/4  "rd_addr_l2"
  Demux/2 -> RAM1/1
  RAM1/2 -> Vector Concatenate/2
  RAM1/1 -> term_2/1
  Demux/3 -> RAM2/1
  RAM2/2 -> Vector Concatenate/3
  RAM2/1 -> term_3/1
  Demux/4 -> RAM3/1
  RAM3/2 -> Vector Concatenate/4
  RAM3/1 -> term_4/1
  Demux/5 -> RAM4/1
  RAM4/2 -> Vector Concatenate/5
  RAM4/1 -> term_5/1
  Demux/6 -> RAM5/1
  RAM5/2 -> Vector Concatenate/6
  RAM5/1 -> term_6/1
  Demux/7 -> RAM6/1
  RAM6/2 -> Vector Concatenate/7
  RAM6/1 -> term_7/1
  Demux/8 -> RAM7/1
  RAM7/2 -> Vector Concatenate/8
  RAM7/1 -> term_8/1
  Demux/9 -> RAM8/1
  RAM8/2 -> Vector Concatenate/9
  RAM8/1 -> term_9/1
  Demux/10 -> RAM9/1
  RAM9/2 -> Vector Concatenate/10
  RAM9/1 -> term_10/1
  Demux/11 -> RAM10/1
  RAM10/2 -> Vector Concatenate/11
  RAM10/1 -> term_11/1
  Demux/12 -> RAM11/1
  RAM11/2 -> Vector Concatenate/12
  RAM11/1 -> term_12/1
  Demux/13 -> RAM12/1
  RAM12/2 -> Vector Concatenate/13
  RAM12/1 -> term_13/1
  Demux/14 -> RAM13/1
  RAM13/2 -> Vector Concatenate/14
  RAM13/1 -> term_14/1
  Demux/15 -> RAM14/1
  RAM14/2 -> Vector Concatenate/15
  RAM14/1 -> term_15/1
  Demux/16 -> RAM15/1
  RAM15/2 -> Vector Concatenate/16
  RAM15/1 -> term_16/1
  Demux/17 -> RAM16/1
  RAM16/2 -> Vector Concatenate/17
  RAM16/1 -> term_17/1
  Demux/18 -> RAM17/1
  RAM17/2 -> Vector Concatenate/18
  RAM17/1 -> term_18/1
  Demux/19 -> RAM18/1
  RAM18/2 -> Vector Concatenate/19
  RAM18/1 -> term_19/1
  Demux/20 -> RAM19/1
  RAM19/2 -> Vector Concatenate/20
  RAM19/1 -> term_20/1
  Demux/21 -> RAM20/1
  RAM20/2 -> Vector Concatenate/21
  RAM20/1 -> term_21/1
  Demux/22 -> RAM21/1
  RAM21/2 -> Vector Concatenate/22
  RAM21/1 -> term_22/1
  Demux/23 -> RAM22/1
  RAM22/2 -> Vector Concatenate/23
  RAM22/1 -> term_23/1
  Demux/24 -> RAM23/1
  RAM23/2 -> Vector Concatenate/24
  RAM23/1 -> term_24/1
  Demux/25 -> RAM24/1
  RAM24/2 -> Vector Concatenate/25
  RAM24/1 -> term_25/1
  Demux/26 -> RAM25/1
  RAM25/2 -> Vector Concatenate/26
  RAM25/1 -> term_26/1
  Demux/27 -> RAM26/1
  RAM26/2 -> Vector Concatenate/27
  RAM26/1 -> term_27/1
  Demux/28 -> RAM27/1
  RAM27/2 -> Vector Concatenate/28
  RAM27/1 -> term_28/1
  Demux/29 -> RAM28/1
  RAM28/2 -> Vector Concatenate/29
  RAM28/1 -> term_29/1
  Demux/30 -> RAM29/1
  RAM29/2 -> Vector Concatenate/30
  RAM29/1 -> term_30/1
  Demux/31 -> RAM30/1
  RAM30/2 -> Vector Concatenate/31
  RAM30/1 -> term_31/1
  Demux/32 -> RAM31/1
  RAM31/2 -> Vector Concatenate/32
  RAM31/1 -> term_32/1
  Demux/33 -> RAM32/1
  RAM32/2 -> Vector Concatenate/33
  RAM32/1 -> term_33/1
  Demux/34 -> RAM33/1
  RAM33/2 -> Vector Concatenate/34
  RAM33/1 -> term_34/1
  Demux/35 -> RAM34/1
  RAM34/2 -> Vector Concatenate/35
  RAM34/1 -> term_35/1
  Demux/36 -> RAM35/1
  RAM35/2 -> Vector Concatenate/36
  RAM35/1 -> term_36/1
  Demux/37 -> RAM36/1
  RAM36/2 -> Vector Concatenate/37
  RAM36/1 -> term_37/1
  Demux/38 -> RAM37/1
  RAM37/2 -> Vector Concatenate/38
  RAM37/1 -> term_38/1
  Demux/39 -> RAM38/1
  RAM38/2 -> Vector Concatenate/39
  RAM38/1 -> term_39/1
  Demux/40 -> RAM39/1
  RAM39/2 -> Vector Concatenate/40
  RAM39/1 -> term_40/1
  Demux/41 -> RAM40/1
  RAM40/2 -> Vector Concatenate/41
  RAM40/1 -> term_41/1
  Demux/42 -> RAM41/1
  RAM41/2 -> Vector Concatenate/42
  RAM41/1 -> term_42/1
  Demux/43 -> RAM42/1
  RAM42/2 -> Vector Concatenate/43
  RAM42/1 -> term_43/1
  Demux/44 -> RAM43/1
  RAM43/2 -> Vector Concatenate/44
  RAM43/1 -> term_44/1
  Demux/45 -> RAM44/1
  RAM44/2 -> Vector Concatenate/45
  RAM44/1 -> term_45/1
  Demux/46 -> RAM45/1
  RAM45/2 -> Vector Concatenate/46
  RAM45/1 -> term_46/1
  Demux/47 -> RAM46/1
  RAM46/2 -> Vector Concatenate/47
  RAM46/1 -> term_47/1
  Demux/48 -> RAM47/1
  RAM47/2 -> Vector Concatenate/48
  RAM47/1 -> term_48/1
  Demux/49 -> RAM48/1
  RAM48/2 -> Vector Concatenate/49
  RAM48/1 -> term_49/1
  Demux/50 -> RAM49/1
  RAM49/2 -> Vector Concatenate/50
  RAM49/1 -> term_50/1
  Demux/51 -> RAM50/1
  RAM50/2 -> Vector Concatenate/51
  RAM50/1 -> term_51/1
  Demux/52 -> RAM51/1
  RAM51/2 -> Vector Concatenate/52
  RAM51/1 -> term_52/1
  Demux/53 -> RAM52/1
  RAM52/2 -> Vector Concatenate/53
  RAM52/1 -> term_53/1
  Demux/54 -> RAM53/1
  RAM53/2 -> Vector Concatenate/54
  RAM53/1 -> term_54/1
  Demux/55 -> RAM54/1
  RAM54/2 -> Vector Concatenate/55
  RAM54/1 -> term_55/1
  Demux/56 -> RAM55/1
  RAM55/2 -> Vector Concatenate/56
  RAM55/1 -> term_56/1
  Demux/57 -> RAM56/1
  RAM56/2 -> Vector Concatenate/57
  RAM56/1 -> term_57/1
  Demux/58 -> RAM57/1
  RAM57/2 -> Vector Concatenate/58
  RAM57/1 -> term_58/1
  Demux/59 -> RAM58/1
  RAM58/2 -> Vector Concatenate/59
  RAM58/1 -> term_59/1
  Demux/60 -> RAM59/1
  RAM59/2 -> Vector Concatenate/60
  RAM59/1 -> term_60/1
  Demux/61 -> RAM60/1
  RAM60/2 -> Vector Concatenate/61
  RAM60/1 -> term_61/1
  Demux/62 -> RAM61/1
  RAM61/2 -> Vector Concatenate/62
  RAM61/1 -> term_62/1
  Demux/63 -> RAM62/1
  RAM62/2 -> Vector Concatenate/63
  RAM62/1 -> term_63/1
  Demux/64 -> RAM63/1
  RAM63/2 -> Vector Concatenate/64
  RAM63/1 -> term_64/1
  rd_row_idx/1 -> Delay1/1
  Delay1/1 -> Terminator1/1

== system model_cnn/HDL CNN Model/Conv Layer 2/Filter Matrix Multiplier1 ==
  note: 1
  note: 2
  note: 3
  note: 4
  note: 5
  note: 6
  note: 7
  note: 8
  note: 9
  note: 10
  note: 11
  note: 12
  note: 13
  note: 14
  note: 15
  note: 16
  samplesIn : Inport
  validIn : Inport  Port=2
  Delay : Delay  DelayLength=1
  Delay1 : Delay  DelayLength=1
  ParallelMACs 0 : Subsystem  mask{filter_dim=1}
      mask prompts: filter_dim "Filter Dimensions"
  ParallelMACs 1 : Subsystem  mask{filter_dim=2}
      mask prompts: filter_dim "Filter Dimensions"
  ParallelMACs 10 : Subsystem  mask{filter_dim=11}
      mask prompts: filter_dim "Filter Dimensions"
  ParallelMACs 11 : Subsystem  mask{filter_dim=12}
      mask prompts: filter_dim "Filter Dimensions"
  ParallelMACs 12 : Subsystem  mask{filter_dim=13}
      mask prompts: filter_dim "Filter Dimensions"
  ParallelMACs 13 : Subsystem  mask{filter_dim=14}
      mask prompts: filter_dim "Filter Dimensions"
  ParallelMACs 14 : Subsystem  mask{filter_dim=15}
      mask prompts: filter_dim "Filter Dimensions"
  ParallelMACs 15 : Subsystem  mask{filter_dim=16}
      mask prompts: filter_dim "Filter Dimensions"
  ParallelMACs 2 : Subsystem  mask{filter_dim=3}
      mask prompts: filter_dim "Filter Dimensions"
  ParallelMACs 3 : Subsystem  mask{filter_dim=4}
      mask prompts: filter_dim "Filter Dimensions"
  ParallelMACs 4 : Subsystem  mask{filter_dim=5}
      mask prompts: filter_dim "Filter Dimensions"
  ParallelMACs 5 : Subsystem  mask{filter_dim=6}
      mask prompts: filter_dim "Filter Dimensions"
  ParallelMACs 6 : Subsystem  mask{filter_dim=7}
      mask prompts: filter_dim "Filter Dimensions"
  ParallelMACs 7 : Subsystem  mask{filter_dim=8}
      mask prompts: filter_dim "Filter Dimensions"
  ParallelMACs 8 : Subsystem  mask{filter_dim=9}
      mask prompts: filter_dim "Filter Dimensions"
  ParallelMACs 9 : Subsystem  mask{filter_dim=10}
      mask prompts: filter_dim "Filter Dimensions"
  Terminator{1..15} (15 alike) : Terminator
  Vector Concatenate : Concatenate  NumInputs=16
  vectorOut : Outport
  validOut : Outport  Port=2
  wires:
  samplesIn/1 -> Delay/1  "samplesIn"
  ParallelMACs 0/2(validOut) -> validOut/1  "vectorOutValid_c2"
  ParallelMACs 1/2(validOut) -> Terminator4/1
  ParallelMACs 1/1(samplesOut) -> Vector Concatenate/2
  ParallelMACs 2/1(samplesOut) -> Vector Concatenate/3
  ParallelMACs 3/1(samplesOut) -> Vector Concatenate/4
  ParallelMACs 4/1(samplesOut) -> Vector Concatenate/5
  ParallelMACs 5/1(samplesOut) -> Vector Concatenate/6
  ParallelMACs 6/1(samplesOut) -> Vector Concatenate/7
  ParallelMACs 7/1(samplesOut) -> Vector Concatenate/8
  ParallelMACs 8/1(samplesOut) -> Vector Concatenate/9
  ParallelMACs 9/1(samplesOut) -> Vector Concatenate/10
  ParallelMACs 10/1(samplesOut) -> Vector Concatenate/11
  ParallelMACs 11/1(samplesOut) -> Vector Concatenate/12
  ParallelMACs 12/1(samplesOut) -> Vector Concatenate/13
  ParallelMACs 14/1(samplesOut) -> Vector Concatenate/15
  ParallelMACs 15/1(samplesOut) -> Vector Concatenate/16
  Vector Concatenate/1 -> vectorOut/1  "vectorOut"
  ParallelMACs 0/1(samplesOut) -> Vector Concatenate/1  "samplesOut_c2"
  ParallelMACs 13/1(samplesOut) -> Vector Concatenate/14
  validIn/1 -> Delay1/1  "samplesInValid"
  Delay/1 -> ParallelMACs 0/1(vectorIn), ParallelMACs 1/1(vectorIn), ParallelMACs 2/1(vectorIn), ParallelMACs 3/1(vectorIn), ParallelMACs 4/1(vectorIn), ParallelMACs 5/1(vectorIn), ParallelMACs 6/1(vectorIn), ParallelMACs 7/1(vectorIn), ParallelMACs 8/1(vectorIn), ParallelMACs 9/1(vectorIn), ParallelMACs 10/1(vectorIn), ParallelMACs 11/1(vectorIn), ParallelMACs 12/1(vectorIn), ParallelMACs 13/1(vectorIn), ParallelMACs 15/1(vectorIn), ParallelMACs 14/1(vectorIn)  "vectorIn_c2"
  Delay1/1 -> ParallelMACs 0/2(validIn), ParallelMACs 1/2(validIn), ParallelMACs 2/2(validIn), ParallelMACs 3/2(validIn), ParallelMACs 4/2(validIn), ParallelMACs 5/2(validIn), ParallelMACs 6/2(validIn), ParallelMACs 7/2(validIn), ParallelMACs 8/2(validIn), ParallelMACs 9/2(validIn), ParallelMACs 10/2(validIn), ParallelMACs 11/2(validIn), ParallelMACs 12/2(validIn), ParallelMACs 13/2(validIn), ParallelMACs 15/2(validIn), ParallelMACs 14/2(validIn)  "validIn_c2"
  ParallelMACs 2/2(validOut) -> Terminator1/1
  ParallelMACs 3/2(validOut) -> Terminator2/1
  ParallelMACs 4/2(validOut) -> Terminator3/1
  ParallelMACs 5/2(validOut) -> Terminator5/1
  ParallelMACs 6/2(validOut) -> Terminator6/1
  ParallelMACs 7/2(validOut) -> Terminator7/1
  ParallelMACs 8/2(validOut) -> Terminator8/1
  ParallelMACs 9/2(validOut) -> Terminator9/1
  ParallelMACs 10/2(validOut) -> Terminator10/1
  ParallelMACs 11/2(validOut) -> Terminator11/1
  ParallelMACs 12/2(validOut) -> Terminator12/1
  ParallelMACs 13/2(validOut) -> Terminator13/1
  ParallelMACs 14/2(validOut) -> Terminator14/1
  ParallelMACs 15/2(validOut) -> Terminator15/1
